simulink model "KugleModel"  (R2018a)
settings: Solver=VariableStepAuto  StartTime=0.0  StopTime=25  FixedStep=1e-3  MaxStep=1e-2  RelTol=1e-5
PreLoadFcn:
  | modelDir = fileparts(get_param(bdroot, 'FileName'));
  | addpath(fullfile(modelDir,'../../Parameters'));
  | addpath(fullfile(modelDir,'../../Model/generated'));
  | addpath(fullfile(modelDir,'../../Misc'));
  | 
  | Parameters_Simulation
  | Constants_Kugle
  | Constants_nominal
InitFcn:
  | Parameters_Simulation
  | Constants_Kugle
  | Constants_nominal
undefined symbols (not defined in the file or in its folder): COM, constants, max_output_torque, x_init
settings Model: Creator=Thomas  LastModifiedBy=Thomas
settings DebuggingCC: UniqueDataStoreMsg=error
settings HardwareCC: ProdBitPerPointer=32  ProdBitPerSizeT=32  ProdBitPerPtrDiffT=32  ProdLargestAtomicInteger=Long  ProdLargestAtomicFloat=Double  ProdWordSize=32  ProdHWDeviceType=ARM Compatible->ARM Cortex
settings ModelReferenceCC: ModelReferenceMinAlgLoopOccurrences=on
settings RTWCC: GenCodeOnly=on  Toolchain=GNU Tools for ARM Embedded Processors
settings GRTTargetCC: TargetLangStandard=C89/C90 (ANSI)  CodeReplacementLibrary=ARM Cortex-M (CMSIS)

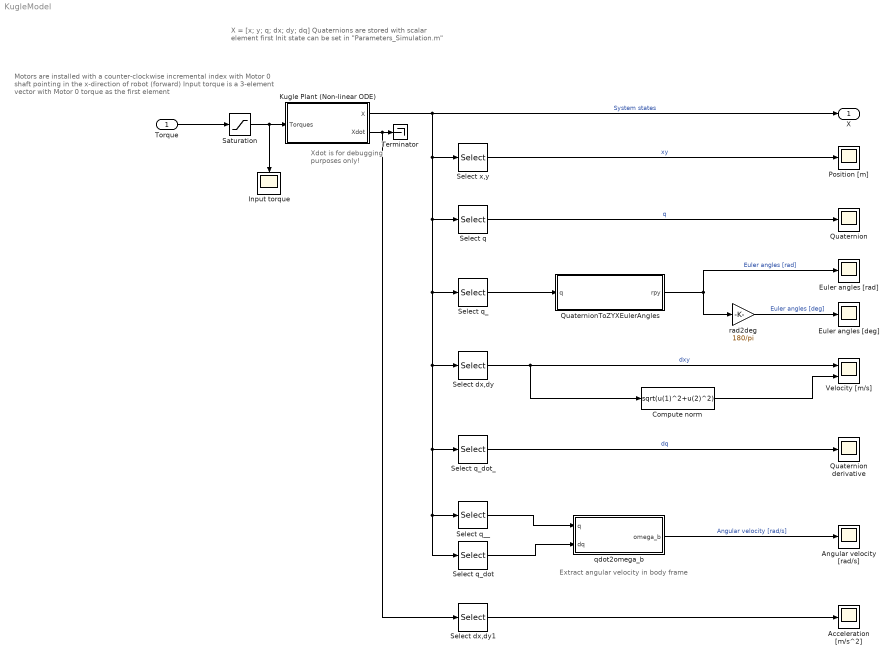
== system KugleModel ==
  note: Xdot is for debugging
      | purposes only!
  note: Motors are installed with a counter-clockwise incremental index with
      | Motor 0 shaft pointing in the x-direction of robot (forward)
      |
      | Input torque is a 3-element vector with Motor 0 torque as the first element
  note: X = [x; y; q; dx; dy; dq]
      | Quaternions are stored with scalar element first
      | Init state can be set in "Parameters_Simulation.m"
  note: Extract angular velocity in body frame
  Torque : Inport  PortDimensions=3
  Acceleration [m/s^2] : Scope
  Angular velocity [rad/s] : Scope
  Compute norm : Fcn  Expr=sqrt(u(1)^2+u(2)^2)
  Euler angles [deg] : Scope
  Euler angles [rad] : Scope
  Input torque : Scope
  Kugle Plant (Non-linear ODE) : Subsystem
  Position [m] : Scope
  Quaternion : Scope
  Quaternion derivative : Scope
  QuaternionToZYXEulerAngles : MATLAB Function  TreatAsAtomicUnit=on
  Saturation : Saturate  UpperLimit=max_output_torque  LowerLimit=-max_output_torque
  Select dx,dy : Selector  InputPortWidth=12  IndexOptions=Index vector (dialog)  Indices=[7,8]  OutputSizes=1
  Select dx,dy1 : Selector  InputPortWidth=12  IndexOptions=Index vector (dialog)  Indices=[7,8]  OutputSizes=1
  Select q : Selector  InputPortWidth=12  IndexOptions=Index vector (dialog)  Indices=[3,4,5,6]  OutputSizes=1
  Select q_ : Selector  InputPortWidth=12  IndexOptions=Index vector (dialog)  Indices=[3,4,5,6]  OutputSizes=1
  Select q__ : Selector  InputPortWidth=12  IndexOptions=Index vector (dialog)  Indices=[3,4,5,6]  OutputSizes=1
  Select q_dot : Selector  InputPortWidth=12  IndexOptions=Index vector (dialog)  Indices=[9,10,11,12]  OutputSizes=1
  Select q_dot_ : Selector  InputPortWidth=12  IndexOptions=Index vector (dialog)  Indices=[9,10,11,12]  OutputSizes=1
  Select x,y : Selector  InputPortWidth=12  IndexOptions=Index vector (dialog)  Indices=[1,2]  OutputSizes=1
  Terminator : Terminator
  Velocity [m/s] : Scope  NumInputPorts=2
  qdot2omega_b : MATLAB Function  TreatAsAtomicUnit=on
  rad2deg : Gain  Gain=180/pi
  X : Outport
  wires:
  Saturation/1 -> Input torque/1, Kugle Plant (Non-linear ODE)/1(Torques)
  Kugle Plant (Non-linear ODE)/1(X) -> Select x,y/1, Select q__/1, Select q_dot/1, Select q_dot_/1, Select dx,dy/1, Select q_/1, Select q/1, X/1  "System states"
  Select q/1 -> Quaternion/1  "q"
  Select q_dot/1 -> qdot2omega_b/2(dq)
  qdot2omega_b/1(omega_b) -> Angular velocity [rad/s]/1  "Angular velocity [rad/s]"
  Select q_dot_/1 -> Quaternion derivative/1  "dq"
  Select dx,dy/1 -> Compute norm/1, Velocity [m/s]/1  "dxy"
  Select x,y/1 -> Position [m]/1  "xy"
  QuaternionToZYXEulerAngles/1(rpy) -> rad2deg/1, Euler angles [rad]/1  "Euler angles [rad]"
  Select q_/1 -> QuaternionToZYXEulerAngles/1(q)
  Kugle Plant (Non-linear ODE)/2(Xdot) -> Select dx,dy1/1, Terminator/1
  Torque/1 -> Saturation/1
  rad2deg/1 -> Euler angles [deg]/1  "Euler angles [deg]"
  Select q__/1 -> qdot2omega_b/1(q)
  Select dx,dy1/1 -> Acceleration [m/s^2]/1
  Compute norm/1 -> Velocity [m/s]/2

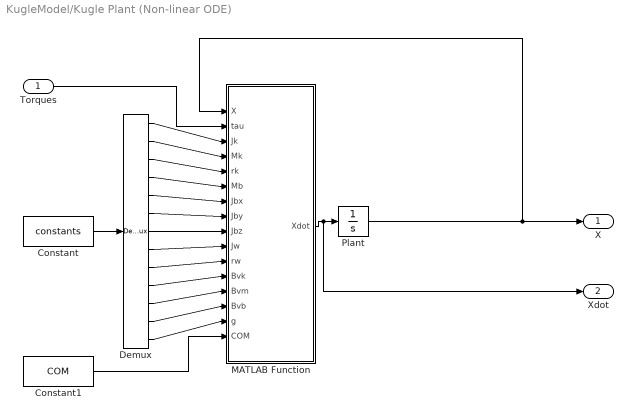
== system KugleModel/Kugle Plant (Non-linear ODE) ==
  Torques : Inport
  Constant : Constant  Value=constants
  Constant1 : Constant  Value=COM
  Demux : Demux  Outputs=13
  MATLAB Function : MATLAB Function  TreatAsAtomicUnit=on
  Plant : Integrator  InitialCondition=x_init
  X : Outport
  Xdot : Outport  Port=2
  wires:
  Demux/12 -> MATLAB Function/14(Bvb)
  Demux/11 -> MATLAB Function/13(Bvm)
  Demux/5 -> MATLAB Function/7(Jbx)
  Demux/8 -> MATLAB Function/10(Jw)
  Demux/1 -> MATLAB Function/3(Jk)
  Constant/1 -> Demux/1
  Demux/3 -> MATLAB Function/5(rk)
  Demux/6 -> MATLAB Function/8(Jby)
  Demux/7 -> MATLAB Function/9(Jbz)
  Demux/10 -> MATLAB Function/12(Bvk)
  Demux/2 -> MATLAB Function/4(Mk)
  Demux/9 -> MATLAB Function/11(rw)
  Demux/4 -> MATLAB Function/6(Mb)
  Torques/1 -> MATLAB Function/2(tau)
  Plant/1 -> MATLAB Function/1(X), X/1
  MATLAB Function/1(Xdot) -> Plant/1, Xdot/1
  Constant1/1 -> MATLAB Function/16(COM)
  Demux/13 -> MATLAB Function/15(g)

== matlab function KugleModel/QuaternionToZYXEulerAngles ==
  data: q input; rpy output
function rpy = Quaternion2ZYXEulerAngles(q)
    rpy = Quaternion2ZYXEulerAngles(q);
end

== matlab function KugleModel/Kugle Plant (Non-linear ODE)/MATLAB Function ==
  data: Xdot output size=12; X input size=12; tau input size=3; Jk input; Mk input; rk input; Mb input; Jbx input; Jby input; Jbz input; Jw input; rw input; Bvk input; Bvm input; Bvb input; g input; COM input size=3
function Xdot = Kugle_ODE(X,tau,Jk,Mk,rk,Mb,Jbx,Jby,Jbz,Jw,rw,Bvk,Bvm,Bvb,g,COM)

beta = 1; % regularization enabled for ODE (plant)

x = X(1);
y = X(2);
q1 = X(3);
q2 = X(4);
q3 = X(5);
q4 = X(6);

dx = X(7);
dy = X(8);
dq1 = X(9);
dq2 = X(10);
dq3 = X(11);
dq4 = X(12);

dchi = reshape(X(7:12), 6, 1);

COM_X = COM(1);
COM_Y = COM(2);
COM_Z = COM(3);

M = mass(COM_X,COM_Y,COM_Z,Jbx,Jby,Jbz,Jk,Jw,Mb,Mk,q1,q2,q3,q4,rk,rw);
C = coriolis(COM_X,COM_Y,COM_Z,Jbx,Jby,Jbz,Jw,Mb,beta,dq1,dq2,dq3,dq4,dx,dy,q1,q2,q3,q4,rk,rw);
G = gravity(COM_X,COM_Y,COM_Z,Mb,beta,g,q1,q2,q3,q4);
D = friction(Bvb,Bvk,Bvm,beta,dq1,dq2,dq3,dq4,dx,dy,q1,q2,q3,q4,rk,rw);
Q = input_forces(q1,q2,q3,q4,rk,rw);


ddchi = M \ (-C*dchi - G - D + Q*tau);

Xdot = [dchi; ddchi];

== matlab function KugleModel/qdot2omega_b ==
  data: q input; omega_b output; dq input
function omega_b = qdot2omega_b(q, dq)
    omega_b = qdot2omega_b(q, dq);
end
